simulink model "eovsa_corr_300mhz"  (R2012b)
settings: Solver=VariableStepDiscrete  SolverMode=SingleTasking  StartTime=0.0  StopTime=5000  RelTol=1e-3
undefined symbols (not defined in the file or in its folder): A, B, gcbh, PCIN, sfp, xlBlockLoadCallback, xlipgetpartsetting
libraries: xbsIndex_r4 x5996, casper_library_misc x52, simulink x33, dspsigops x24, xps_library x15, casper_library_delays x2
(part 21 of 65)

== system eovsa_corr_300mhz/pfb_fft/power_td1 ==
  note: The dsp48_sq_add block is a stack of cascaded DSP48 slices.
      | It replaces a previous less efficient implementation that used
      | multipliers followed by an adder tree.  There is more room for
      | optimization here (e.g. by including the accumulation(s) in the
      | stack(s) of cascaded DSP48 slices, but the current (interim)
      | implementation was done to avoid having to change any
      | control logic.
      |
      | The overall latency of the dsp48_sq_add block is 2 cycles
      | longer than the original multipler/adder implementation.
      | To accomodate this change in latency, the sync_in signal
      | has been delayed by a corresponding 2 cycles.
  sync : Inport
  din : Inport  Port=2
  acc_len : Inport  Port=3
  acc_start_skip : Inport  Port=4
  Accumulator2 : xbsIndex_r4/Accumulator  operation=Add  n_bits=48  overflow=Wrap  scale=1  rst=on  infoeditControl=reset for floating point data type must be asserted for a minimum of 2 cycles  hasbypass=off  en=on  latency=0  dbl_ovrd=off  msb_inp=100  msb=100  lsb=-100  use_behavioral_HDL=on  implementation=Fabric  block_type=accum
      settings: block_version=11.4
  Accumulator3 : xbsIndex_r4/Accumulator  operation=Add  n_bits=64  overflow=Wrap  scale=1  rst=on  infoeditControl=reset for floating point data type must be asserted for a minimum of 2 cycles  hasbypass=off  en=on  latency=0  dbl_ovrd=off  msb_inp=100  msb=100  lsb=-100  use_behavioral_HDL=on  implementation=Fabric  block_type=accum
      settings: block_version=11.4
  Accumulator4 : xbsIndex_r4/Accumulator  operation=Add  n_bits=32  overflow=Wrap  scale=1  rst=on  infoeditControl=reset for floating point data type must be asserted for a minimum of 2 cycles  hasbypass=on  en=off  latency=0  dbl_ovrd=off  msb_inp=100  msb=100  lsb=-100  use_behavioral_HDL=off  implementation=DSP48  block_type=accum
      settings: block_version=11.4
  AddSub3 : xbsIndex_r4/AddSub  mode=Addition  use_carryin=off  use_carryout=off  en=off  latency=1  precision=User Defined  arith_type=Unsigned  n_bits=16  bin_pt=0  quantization=Truncate  overflow=Wrap  dbl_ovrd=off  use_behavioral_HDL=on  hw_selection=DSP48  pipelined=off  block_type=addsub
  AddSub4 : xbsIndex_r4/AddSub  mode=Subtraction  use_carryin=off  use_carryout=off  en=off  latency=1  precision=User Defined  arith_type=Unsigned  n_bits=16  bin_pt=0  quantization=Truncate  overflow=Wrap  dbl_ovrd=off  use_behavioral_HDL=on  hw_selection=DSP48  pipelined=off  block_type=addsub
  Constant : xbsIndex_r4/Constant  const=0  gui_display_data_type=Fixed-point  arith_type=Unsigned  n_bits=32  bin_pt=14  preci_type=Single  exp_width=8  frac_width=24  explicit_period=on  period=1  equ=P=C  opselect=C  inp2=PCIN>>17  opr=+  inp1=P  carry=CIN  dbl_ovrd=off  block_type=constant
      settings: block_version=11.4
  Constant1 : xbsIndex_r4/Constant  const=1  gui_display_data_type=Fixed-point  arith_type=Unsigned  n_bits=1  bin_pt=0  preci_type=Single  exp_width=8  frac_width=24  explicit_period=on  period=1  equ=P=C  opselect=C  inp2=PCIN>>17  opr=+  inp1=P  carry=CIN  dbl_ovrd=off  block_type=constant
      settings: block_version=11.4
  Convert1 : xbsIndex_r4/Convert  gui_display_data_type=Fixed-point  arith_type=Unsigned  n_bits=64  bin_pt=18  float_type=Single  exp_bits=8  fraction_bits=24  quantization=Truncate  overflow=Wrap  en=off  latency=0  dbl_ovrd=off  pipeline=off  block_type=convert
      settings: block_version=11.4
  Convert2 : xbsIndex_r4/Convert  gui_display_data_type=Fixed-point  arith_type=Unsigned  n_bits=64  bin_pt=18  float_type=Single  exp_bits=8  fraction_bits=24  quantization=Truncate  overflow=Wrap  en=off  latency=0  dbl_ovrd=off  pipeline=off  block_type=convert
      settings: block_version=11.4
  Convert3 : xbsIndex_r4/Convert  gui_display_data_type=Fixed-point  arith_type=Unsigned  n_bits=32  bin_pt=14  float_type=Single  exp_bits=8  fraction_bits=24  quantization=Truncate  overflow=Wrap  en=off  latency=0  dbl_ovrd=off  pipeline=off  block_type=convert
      settings: block_version=11.4
  Convert4 : xbsIndex_r4/Convert  gui_display_data_type=Fixed-point  arith_type=Unsigned  n_bits=1  bin_pt=0  float_type=Single  exp_bits=8  fraction_bits=24  quantization=Truncate  overflow=Wrap  en=off  latency=0  dbl_ovrd=off  pipeline=off  block_type=convert
      settings: block_version=11.4
  Convert5 : xbsIndex_r4/Convert  gui_display_data_type=Fixed-point  arith_type="Signed  (2's comp)"  n_bits=34  bin_pt=14  float_type=Single  exp_bits=8  fraction_bits=24  quantization=Truncate  overflow=Wrap  en=off  latency=0  dbl_ovrd=off  pipeline=on  block_type=convert
      settings: block_version=11.4
  Counter : xbsIndex_r4/Counter  cnt_type=Free Running  cnt_to=0  operation=Up  start_count=0  cnt_by_val=1  arith_type=Unsigned  n_bits=16  bin_pt=0  load_pin=off  rst=on  en=on  explicit_period=off  period=1  dbl_ovrd=off  use_behavioral_HDL=off  implementation=Fabric  block_type=counter
      settings: block_version=11.4
  Counter1 : xbsIndex_r4/Counter  cnt_type=Free Running  cnt_to=3000  operation=Up  start_count=0  cnt_by_val=1  arith_type=Unsigned  n_bits=32  bin_pt=0  load_pin=off  rst=off  en=on  explicit_period=on  period=1  dbl_ovrd=off  use_behavioral_HDL=on  implementation=Fabric  block_type=counter
      settings: block_version=11.4
  Delay{1,6,9,23} (4 alike) : xbsIndex_r4/Delay  rst=off  infoeditControl=Selection of Reset will increase slice count due to use of real FFs and instead of SRLs  en=off  latency=5  dbl_ovrd=off  reg_retiming=on  block_type=delay
      settings: block_version=11.4
  Delay{2..4,8,10..14,16,18,22,25} (13 alike) : xbsIndex_r4/Delay  rst=off  infoeditControl=Selection of Reset will increase slice count due to use of real FFs and instead of SRLs  en=off  latency=1  dbl_ovrd=off  reg_retiming=on  block_type=delay
      settings: block_version=11.4
  Delay15 : xbsIndex_r4/Delay  rst=off  infoeditControl=Selection of Reset will increase slice count due to use of real FFs and instead of SRLs  en=off  latency=1  dbl_ovrd=off  reg_retiming=off  block_type=delay
      settings: block_version=11.4
  Delay{7,17,19..21} (5 alike) : xbsIndex_r4/Delay  rst=off  infoeditControl=Selection of Reset will increase slice count due to use of real FFs and instead of SRLs  en=off  latency=2  dbl_ovrd=off  reg_retiming=on  block_type=delay
      settings: block_version=11.4
  Delay24 : xbsIndex_r4/Delay  rst=off  infoeditControl=Selection of Reset will increase slice count due to use of real FFs and instead of SRLs  en=off  latency=9  dbl_ovrd=off  reg_retiming=on  block_type=delay
      settings: block_version=11.4
  Delay5 : xbsIndex_r4/Delay  rst=off  infoeditControl=Selection of Reset will increase slice count due to use of real FFs and instead of SRLs  en=off  latency=3  dbl_ovrd=off  reg_retiming=on  block_type=delay
      settings: block_version=11.4
  Logical1 : xbsIndex_r4/Logical  logical_function=XOR  inputs=2  en=off  latency=1  precision=Full  arith_type=Unsigned  n_bits=16  bin_pt=0  align_bp=on  dbl_ovrd=off  block_type=logical
      settings: block_version=11.4
  Mux : xbsIndex_r4/Mux  inputs=2  en=off  latency=1  precision=Full  arith_type=Unsigned  n_bits=16  bin_pt=14  quantization=Truncate  overflow=Wrap  dbl_ovrd=off  block_type=mux
      settings: block_version=11.4
  Reinterpret : xbsIndex_r4/Reinterpret  force_arith_type=on  arith_type=Unsigned  force_bin_pt=on  bin_pt=0  block_type=reinterpret
      settings: infoedit="Changes signal type without altering the binary representation.   You can changed the signal between signed and unsigned, and relocate the binary point.<br><br>Hardware notes: In hardware this block costs nothing.<br><br>Example:  Suppose the input is 6 bits wide, signed, with 2 fractional bits, and the output is forced to unsigned with 0 fractional bits.  Then an input of -2.0 (1110.00 in binary 2's complement) becomes an output of 56 (111000 in binary)."
  Reinterpret1 : xbsIndex_r4/Reinterpret  force_arith_type=on  arith_type=Unsigned  force_bin_pt=on  bin_pt=0  block_type=reinterpret
      settings: infoedit="Changes signal type without altering the binary representation.   You can changed the signal between signed and unsigned, and relocate the binary point.<br><br>Hardware notes: In hardware this block costs nothing.<br><br>Example:  Suppose the input is 6 bits wide, signed, with 2 fractional bits, and the output is forced to unsigned with 0 fractional bits.  Then an input of -2.0 (1110.00 in binary 2's complement) becomes an output of 56 (111000 in binary)."
  Reinterpret2 : xbsIndex_r4/Reinterpret  force_arith_type=on  arith_type=Unsigned  force_bin_pt=on  bin_pt=18  block_type=reinterpret
  Relational2 : xbsIndex_r4/Relational  mode=a<b  en=off  latency=1  dbl_ovrd=off  block_type=relational
  Relational3 : xbsIndex_r4/Relational  mode=a<b  en=off  latency=1  dbl_ovrd=off  block_type=relational
  Slice1 : xbsIndex_r4/Slice  nbits=32  boolean_output=off  mode=Lower Bit Location + Width  bit1=0  base1=MSB of Input  bit0=13  base0=LSB of Input  dbl_ovrd=off  block_type=slice
  big_square_square : Subsystem  AncestorBlock=casper_library_misc/power_dsp48e  mask(wide_power){bitwidth=17}
      mask prompts: bitwidth "Input bit width:"
      mask help: Computes the power of a wide complex number using 3 DSP48Es.
      mask Display:
      | port_label('input', 1, 'c');
      | port_label('output', 1, 'p');
      | disp(['Z^-', num2str(5)]);
  bus_expand : Subsystem  AncestorBlock=casper_library_flow_control/bus_expand  mask(bus_expand){mode=divisions of equal size, outputNum=4, outputWidth=8, outputBinaryPt=7, outputArithmeticType=1, show_format=off, outputToWorkspace=off, variablePrefix=out, outputToModelAsWell=on}
      mask prompts: outputNum "Number of outputs:"; outputWidth "Output width:"; outputBinaryPt "Output binary point position:"; outputArithmeticType "Output arithmetic type (ufix=0, fix=1, bool=2):"; show_format "Print format string?"; outputToWorkspace "Output to workspace?"; variablePrefix "Variable name prefix:"; outputToModelAsWell "Output to model as well?"
      mask help:
      | Expands a 'bus' made using a bus_create or Xilinx
      | concat block.
      | The input will be divided into the specified number
      | of outputs with the specified arithmetic types.
      | Divisions are made from most significant bit.
      mask init: same as eovsa_corr_300mhz/bus_expand7
      settings: AttributesFormatString=4 outputs
      mask TypeOptions mode: divisions of equal size | divisions of arbitrary size
      mask Callback mode: bus_expand_callback();
      mask Callback outputWidth: bus_expand_callback();
      mask Callback outputToWorkspace: bus_expand_callback();
  dsp48_sq_add : Subsystem
  gen_50_pps : Subsystem  mask{fpga_clk_sub=fpga_clk}
      mask prompts: fpga_clk_sub "FPGA Clock Frequency (MHz)"
  pulse generator skip first : Subsystem  mask{period=2 ^ (fft_size - 1)}
      mask prompts: period "Period (clock cycles)"
  acc_num : Outport
  P : Outport  Port=2
  P2 : Outport  Port=3
  acc_valid : Outport  Port=4
  wires:
  sync/1 -> Delay13/1
  Delay14/1 -> dsp48_sq_add/4(d)
  Delay12/1 -> dsp48_sq_add/3(c)
  Delay11/1 -> dsp48_sq_add/2(b)
  Delay10/1 -> dsp48_sq_add/1(a)
  Constant1/1 -> AddSub4/2
  acc_start_skip/1 -> AddSub4/1
  gen_50_pps/2(sync_out) -> pulse generator skip first/1(sync)
  Delay13/1 -> gen_50_pps/1(sync)
  gen_50_pps/1(50pps) -> [pps50]
  Delay9/1 -> Accumulator3/3, Accumulator2/3
  Delay23/1 -> Counter1/1, Delay21/1, Accumulator3/2, Accumulator2/2
  Delay24/1 -> Delay23/1
  Delay22/1 -> Delay9/1
  Delay21/1 -> acc_valid/1
  Delay20/1 -> P2/1
  Delay19/1 -> P/1
  Delay7/1 -> acc_num/1
  Delay18/1 -> Delay22/1
  Delay17/1 -> Delay24/1
  Delay16/1 -> Delay1/1
  [pps50] -> Counter/1
  Accumulator3/1 -> Reinterpret1/1
  Convert1/1 -> Accumulator3/1
  big_square_square/1(p) -> Reinterpret2/1
  Slice1/1 -> Delay19/1
  Reinterpret/1 -> Slice1/1
  Convert2/1 -> Accumulator2/1
  [data_valid] -> Delay18/1
  [data] -> Delay15/1, Delay16/1
  Delay6/1 -> Delay8/1, Accumulator4/2
  Delay4/1 -> Delay5/1
  Convert3/1 -> Delay3/1
  Delay2/1 -> Delay6/1
  [reset_frame] -> Delay25/1
  AddSub4/1 -> Relational3/2, AddSub3/1
  Logical1/1 -> Convert4/1
  [data_frame] -> Mux/3
  Constant/1 -> Mux/2
  Convert4/1 -> Delay4/1
  Relational2/1 -> Logical1/2
  Relational3/1 -> Logical1/1
  AddSub3/1 -> Relational2/2
  acc_len/1 -> AddSub3/2
  Counter/1 -> Relational2/1, Relational3/1
  pulse generator skip first/1(pulse) -> [reset_frame], Counter/2
  [pps50] -> Delay17/1
  Delay1/1 -> Convert2/1
  Reinterpret1/1 -> Delay20/1
  Accumulator2/1 -> Reinterpret/1
  Counter1/1 -> Delay7/1
  dsp48_sq_add/1(p) -> Convert3/1
  bus_expand/3(out2) -> Delay12/1
  bus_expand/2(out3) -> Delay11/1
  bus_expand/1(msb_out4) -> Delay10/1
  bus_expand/4(lsb_out1) -> Delay14/1
  din/1 -> bus_expand/1(bus_in)
  Mux/1 -> [data]
  Delay15/1 -> Convert5/1
  Convert5/1 -> big_square_square/1(c)
  Reinterpret2/1 -> Convert1/1
  Delay8/1 -> [data_valid]
  Accumulator4/1 -> [data_frame]
  Delay5/1 -> Mux/1
  Delay3/1 -> Accumulator4/1
  Delay25/1 -> Delay2/1

== system eovsa_corr_300mhz/pfb_fft/power_td2 ==
  note: The dsp48_sq_add block is a stack of cascaded DSP48 slices.
      | It replaces a previous less efficient implementation that used
      | multipliers followed by an adder tree.  There is more room for
      | optimization here (e.g. by including the accumulation(s) in the
      | stack(s) of cascaded DSP48 slices, but the current (interim)
      | implementation was done to avoid having to change any
      | control logic.
      |
      | The overall latency of the dsp48_sq_add block is 2 cycles
      | longer than the original multipler/adder implementation.
      | To accomodate this change in latency, the sync_in signal
      | has been delayed by a corresponding 2 cycles.
  sync : Inport
  din : Inport  Port=2
  acc_len : Inport  Port=3
  acc_start_skip : Inport  Port=4
  Accumulator2 : xbsIndex_r4/Accumulator  operation=Add  n_bits=48  overflow=Wrap  scale=1  rst=on  infoeditControl=reset for floating point data type must be asserted for a minimum of 2 cycles  hasbypass=off  en=on  latency=0  dbl_ovrd=off  msb_inp=100  msb=100  lsb=-100  use_behavioral_HDL=on  implementation=Fabric  block_type=accum
      settings: block_version=11.4
  Accumulator3 : xbsIndex_r4/Accumulator  operation=Add  n_bits=64  overflow=Wrap  scale=1  rst=on  infoeditControl=reset for floating point data type must be asserted for a minimum of 2 cycles  hasbypass=off  en=on  latency=0  dbl_ovrd=off  msb_inp=100  msb=100  lsb=-100  use_behavioral_HDL=on  implementation=Fabric  block_type=accum
      settings: block_version=11.4
  Accumulator4 : xbsIndex_r4/Accumulator  operation=Add  n_bits=32  overflow=Wrap  scale=1  rst=on  infoeditControl=reset for floating point data type must be asserted for a minimum of 2 cycles  hasbypass=on  en=off  latency=0  dbl_ovrd=off  msb_inp=100  msb=100  lsb=-100  use_behavioral_HDL=off  implementation=DSP48  block_type=accum
      settings: block_version=11.4
  AddSub3 : xbsIndex_r4/AddSub  mode=Addition  use_carryin=off  use_carryout=off  en=off  latency=1  precision=User Defined  arith_type=Unsigned  n_bits=16  bin_pt=0  quantization=Truncate  overflow=Wrap  dbl_ovrd=off  use_behavioral_HDL=on  hw_selection=DSP48  pipelined=off  block_type=addsub
  AddSub4 : xbsIndex_r4/AddSub  mode=Subtraction  use_carryin=off  use_carryout=off  en=off  latency=1  precision=User Defined  arith_type=Unsigned  n_bits=16  bin_pt=0  quantization=Truncate  overflow=Wrap  dbl_ovrd=off  use_behavioral_HDL=on  hw_selection=DSP48  pipelined=off  block_type=addsub
  Constant : xbsIndex_r4/Constant  const=0  gui_display_data_type=Fixed-point  arith_type=Unsigned  n_bits=32  bin_pt=14  preci_type=Single  exp_width=8  frac_width=24  explicit_period=on  period=1  equ=P=C  opselect=C  inp2=PCIN>>17  opr=+  inp1=P  carry=CIN  dbl_ovrd=off  block_type=constant
      settings: block_version=11.4
  Constant1 : xbsIndex_r4/Constant  const=1  gui_display_data_type=Fixed-point  arith_type=Unsigned  n_bits=1  bin_pt=0  preci_type=Single  exp_width=8  frac_width=24  explicit_period=on  period=1  equ=P=C  opselect=C  inp2=PCIN>>17  opr=+  inp1=P  carry=CIN  dbl_ovrd=off  block_type=constant
      settings: block_version=11.4
  Convert1 : xbsIndex_r4/Convert  gui_display_data_type=Fixed-point  arith_type=Unsigned  n_bits=64  bin_pt=18  float_type=Single  exp_bits=8  fraction_bits=24  quantization=Truncate  overflow=Wrap  en=off  latency=0  dbl_ovrd=off  pipeline=off  block_type=convert
      settings: block_version=11.4
  Convert2 : xbsIndex_r4/Convert  gui_display_data_type=Fixed-point  arith_type=Unsigned  n_bits=64  bin_pt=18  float_type=Single  exp_bits=8  fraction_bits=24  quantization=Truncate  overflow=Wrap  en=off  latency=0  dbl_ovrd=off  pipeline=off  block_type=convert
      settings: block_version=11.4
  Convert3 : xbsIndex_r4/Convert  gui_display_data_type=Fixed-point  arith_type=Unsigned  n_bits=32  bin_pt=14  float_type=Single  exp_bits=8  fraction_bits=24  quantization=Truncate  overflow=Wrap  en=off  latency=0  dbl_ovrd=off  pipeline=off  block_type=convert
      settings: block_version=11.4
  Convert4 : xbsIndex_r4/Convert  gui_display_data_type=Fixed-point  arith_type=Unsigned  n_bits=1  bin_pt=0  float_type=Single  exp_bits=8  fraction_bits=24  quantization=Truncate  overflow=Wrap  en=off  latency=0  dbl_ovrd=off  pipeline=off  block_type=convert
      settings: block_version=11.4
  Convert5 : xbsIndex_r4/Convert  gui_display_data_type=Fixed-point  arith_type="Signed  (2's comp)"  n_bits=34  bin_pt=14  float_type=Single  exp_bits=8  fraction_bits=24  quantization=Truncate  overflow=Wrap  en=off  latency=0  dbl_ovrd=off  pipeline=on  block_type=convert
      settings: block_version=11.4
  Counter : xbsIndex_r4/Counter  cnt_type=Free Running  cnt_to=0  operation=Up  start_count=0  cnt_by_val=1  arith_type=Unsigned  n_bits=16  bin_pt=0  load_pin=off  rst=on  en=on  explicit_period=off  period=1  dbl_ovrd=off  use_behavioral_HDL=off  implementation=Fabric  block_type=counter
      settings: block_version=11.4
  Counter1 : xbsIndex_r4/Counter  cnt_type=Free Running  cnt_to=3000  operation=Up  start_count=0  cnt_by_val=1  arith_type=Unsigned  n_bits=32  bin_pt=0  load_pin=off  rst=off  en=on  explicit_period=on  period=1  dbl_ovrd=off  use_behavioral_HDL=on  implementation=Fabric  block_type=counter
      settings: block_version=11.4
  Delay{1,6,9,23} (4 alike) : xbsIndex_r4/Delay  rst=off  infoeditControl=Selection of Reset will increase slice count due to use of real FFs and instead of SRLs  en=off  latency=5  dbl_ovrd=off  reg_retiming=on  block_type=delay
      settings: block_version=11.4
  Delay{2..4,8,10..14,16,18,22,25} (13 alike) : xbsIndex_r4/Delay  rst=off  infoeditControl=Selection of Reset will increase slice count due to use of real FFs and instead of SRLs  en=off  latency=1  dbl_ovrd=off  reg_retiming=on  block_type=delay
      settings: block_version=11.4
  Delay15 : xbsIndex_r4/Delay  rst=off  infoeditControl=Selection of Reset will increase slice count due to use of real FFs and instead of SRLs  en=off  latency=1  dbl_ovrd=off  reg_retiming=off  block_type=delay
      settings: block_version=11.4
  Delay{7,17,19..21} (5 alike) : xbsIndex_r4/Delay  rst=off  infoeditControl=Selection of Reset will increase slice count due to use of real FFs and instead of SRLs  en=off  latency=2  dbl_ovrd=off  reg_retiming=on  block_type=delay
      settings: block_version=11.4
  Delay24 : xbsIndex_r4/Delay  rst=off  infoeditControl=Selection of Reset will increase slice count due to use of real FFs and instead of SRLs  en=off  latency=9  dbl_ovrd=off  reg_retiming=on  block_type=delay
      settings: block_version=11.4
  Delay5 : xbsIndex_r4/Delay  rst=off  infoeditControl=Selection of Reset will increase slice count due to use of real FFs and instead of SRLs  en=off  latency=3  dbl_ovrd=off  reg_retiming=on  block_type=delay
      settings: block_version=11.4
  Logical1 : xbsIndex_r4/Logical  logical_function=XOR  inputs=2  en=off  latency=1  precision=Full  arith_type=Unsigned  n_bits=16  bin_pt=0  align_bp=on  dbl_ovrd=off  block_type=logical
      settings: block_version=11.4
  Mux : xbsIndex_r4/Mux  inputs=2  en=off  latency=1  precision=Full  arith_type=Unsigned  n_bits=16  bin_pt=14  quantization=Truncate  overflow=Wrap  dbl_ovrd=off  block_type=mux
      settings: block_version=11.4
  Reinterpret : xbsIndex_r4/Reinterpret  force_arith_type=on  arith_type=Unsigned  force_bin_pt=on  bin_pt=0  block_type=reinterpret
      settings: infoedit="Changes signal type without altering the binary representation.   You can changed the signal between signed and unsigned, and relocate the binary point.<br><br>Hardware notes: In hardware this block costs nothing.<br><br>Example:  Suppose the input is 6 bits wide, signed, with 2 fractional bits, and the output is forced to unsigned with 0 fractional bits.  Then an input of -2.0 (1110.00 in binary 2's complement) becomes an output of 56 (111000 in binary)."
  Reinterpret1 : xbsIndex_r4/Reinterpret  force_arith_type=on  arith_type=Unsigned  force_bin_pt=on  bin_pt=0  block_type=reinterpret
      settings: infoedit="Changes signal type without altering the binary representation.   You can changed the signal between signed and unsigned, and relocate the binary point.<br><br>Hardware notes: In hardware this block costs nothing.<br><br>Example:  Suppose the input is 6 bits wide, signed, with 2 fractional bits, and the output is forced to unsigned with 0 fractional bits.  Then an input of -2.0 (1110.00 in binary 2's complement) becomes an output of 56 (111000 in binary)."
  Reinterpret2 : xbsIndex_r4/Reinterpret  force_arith_type=on  arith_type=Unsigned  force_bin_pt=on  bin_pt=18  block_type=reinterpret
  Relational2 : xbsIndex_r4/Relational  mode=a<b  en=off  latency=1  dbl_ovrd=off  block_type=relational
  Relational3 : xbsIndex_r4/Relational  mode=a<b  en=off  latency=1  dbl_ovrd=off  block_type=relational
  Slice1 : xbsIndex_r4/Slice  nbits=32  boolean_output=off  mode=Lower Bit Location + Width  bit1=0  base1=MSB of Input  bit0=13  base0=LSB of Input  dbl_ovrd=off  block_type=slice
  big_square_square : Subsystem  AncestorBlock=casper_library_misc/power_dsp48e  mask(wide_power){bitwidth=17}
      mask prompts: bitwidth "Input bit width:"
      mask help: Computes the power of a wide complex number using 3 DSP48Es.
      mask Display:
      | port_label('input', 1, 'c');
      | port_label('output', 1, 'p');
      | disp(['Z^-', num2str(5)]);
  bus_expand : Subsystem  AncestorBlock=casper_library_flow_control/bus_expand  mask(bus_expand){mode=divisions of equal size, outputNum=4, outputWidth=8, outputBinaryPt=7, outputArithmeticType=1, show_format=off, outputToWorkspace=off, variablePrefix=out, outputToModelAsWell=on}
      mask prompts: outputNum "Number of outputs:"; outputWidth "Output width:"; outputBinaryPt "Output binary point position:"; outputArithmeticType "Output arithmetic type (ufix=0, fix=1, bool=2):"; show_format "Print format string?"; outputToWorkspace "Output to workspace?"; variablePrefix "Variable name prefix:"; outputToModelAsWell "Output to model as well?"
      mask help:
      | Expands a 'bus' made using a bus_create or Xilinx
      | concat block.
      | The input will be divided into the specified number
      | of outputs with the specified arithmetic types.
      | Divisions are made from most significant bit.
      mask init: same as eovsa_corr_300mhz/bus_expand7
      settings: AttributesFormatString=4 outputs
      mask TypeOptions mode: divisions of equal size | divisions of arbitrary size
      mask Callback mode: bus_expand_callback();
      mask Callback outputWidth: bus_expand_callback();
      mask Callback outputToWorkspace: bus_expand_callback();
  dsp48_sq_add : Subsystem
  gen_50_pps : Subsystem  mask{fpga_clk_sub=fpga_clk}
      mask prompts: fpga_clk_sub "FPGA Clock Frequency (MHz)"
  pulse generator skip first : Subsystem  mask{period=2 ^ (fft_size - 1)}
      mask prompts: period "Period (clock cycles)"
  acc_num : Outport
  P : Outport  Port=2
  P2 : Outport  Port=3
  acc_valid : Outport  Port=4
  wires:
  Delay25/1 -> Delay2/1
  Delay3/1 -> Accumulator4/1
  Delay5/1 -> Mux/1
  Accumulator4/1 -> [data_frame]
  Delay8/1 -> [data_valid]
  Reinterpret2/1 -> Convert1/1
  Convert5/1 -> big_square_square/1(c)
  Delay15/1 -> Convert5/1
  Mux/1 -> [data]
  din/1 -> bus_expand/1(bus_in)
  bus_expand/4(lsb_out1) -> Delay14/1
  bus_expand/1(msb_out4) -> Delay10/1
  bus_expand/2(out3) -> Delay11/1
  bus_expand/3(out2) -> Delay12/1
  dsp48_sq_add/1(p) -> Convert3/1
  Counter1/1 -> Delay7/1
  Accumulator2/1 -> Reinterpret/1
  Reinterpret1/1 -> Delay20/1
  Delay1/1 -> Convert2/1
  [pps50] -> Delay17/1
  pulse generator skip first/1(pulse) -> Counter/2, [reset_frame]
  Counter/1 -> Relational3/1, Relational2/1
  acc_len/1 -> AddSub3/2
  AddSub3/1 -> Relational2/2
  Relational3/1 -> Logical1/1
  Relational2/1 -> Logical1/2
  Convert4/1 -> Delay4/1
  Constant/1 -> Mux/2
  [data_frame] -> Mux/3
  Logical1/1 -> Convert4/1
  AddSub4/1 -> AddSub3/1, Relational3/2
  [reset_frame] -> Delay25/1
  Delay2/1 -> Delay6/1
  Convert3/1 -> Delay3/1
  Delay4/1 -> Delay5/1
  Delay6/1 -> Accumulator4/2, Delay8/1
  [data] -> Delay16/1, Delay15/1
  [data_valid] -> Delay18/1
  Convert2/1 -> Accumulator2/1
  Reinterpret/1 -> Slice1/1
  Slice1/1 -> Delay19/1
  big_square_square/1(p) -> Reinterpret2/1
  Convert1/1 -> Accumulator3/1
  Accumulator3/1 -> Reinterpret1/1
  [pps50] -> Counter/1
  Delay16/1 -> Delay1/1
  Delay17/1 -> Delay24/1
  Delay18/1 -> Delay22/1
  Delay7/1 -> acc_num/1
  Delay19/1 -> P/1
  Delay20/1 -> P2/1
  Delay21/1 -> acc_valid/1
  Delay22/1 -> Delay9/1
  Delay24/1 -> Delay23/1
  Delay23/1 -> Accumulator2/2, Accumulator3/2, Delay21/1, Counter1/1
  Delay9/1 -> Accumulator2/3, Accumulator3/3
  gen_50_pps/1(50pps) -> [pps50]
  Delay13/1 -> gen_50_pps/1(sync)
  gen_50_pps/2(sync_out) -> pulse generator skip first/1(sync)
  acc_start_skip/1 -> AddSub4/1
  Constant1/1 -> AddSub4/2
  Delay10/1 -> dsp48_sq_add/1(a)
  Delay11/1 -> dsp48_sq_add/2(b)
  Delay12/1 -> dsp48_sq_add/3(c)
  Delay14/1 -> dsp48_sq_add/4(d)
  sync/1 -> Delay13/1

== system eovsa_corr_300mhz/pfb_fft/power_td3 ==
  note: The dsp48_sq_add block is a stack of cascaded DSP48 slices.
      | It replaces a previous less efficient implementation that used
      | multipliers followed by an adder tree.  There is more room for
      | optimization here (e.g. by including the accumulation(s) in the
      | stack(s) of cascaded DSP48 slices, but the current (interim)
      | implementation was done to avoid having to change any
      | control logic.
      |
      | The overall latency of the dsp48_sq_add block is 2 cycles
      | longer than the original multipler/adder implementation.
      | To accomodate this change in latency, the sync_in signal
      | has been delayed by a corresponding 2 cycles.
  sync : Inport
  din : Inport  Port=2
  acc_len : Inport  Port=3
  acc_start_skip : Inport  Port=4
  Accumulator2 : xbsIndex_r4/Accumulator  operation=Add  n_bits=48  overflow=Wrap  scale=1  rst=on  infoeditControl=reset for floating point data type must be asserted for a minimum of 2 cycles  hasbypass=off  en=on  latency=0  dbl_ovrd=off  msb_inp=100  msb=100  lsb=-100  use_behavioral_HDL=on  implementation=Fabric  block_type=accum
      settings: block_version=11.4
  Accumulator3 : xbsIndex_r4/Accumulator  operation=Add  n_bits=64  overflow=Wrap  scale=1  rst=on  infoeditControl=reset for floating point data type must be asserted for a minimum of 2 cycles  hasbypass=off  en=on  latency=0  dbl_ovrd=off  msb_inp=100  msb=100  lsb=-100  use_behavioral_HDL=on  implementation=Fabric  block_type=accum
      settings: block_version=11.4
  Accumulator4 : xbsIndex_r4/Accumulator  operation=Add  n_bits=32  overflow=Wrap  scale=1  rst=on  infoeditControl=reset for floating point data type must be asserted for a minimum of 2 cycles  hasbypass=on  en=off  latency=0  dbl_ovrd=off  msb_inp=100  msb=100  lsb=-100  use_behavioral_HDL=off  implementation=DSP48  block_type=accum
      settings: block_version=11.4
  AddSub3 : xbsIndex_r4/AddSub  mode=Addition  use_carryin=off  use_carryout=off  en=off  latency=1  precision=User Defined  arith_type=Unsigned  n_bits=16  bin_pt=0  quantization=Truncate  overflow=Wrap  dbl_ovrd=off  use_behavioral_HDL=on  hw_selection=DSP48  pipelined=off  block_type=addsub
  AddSub4 : xbsIndex_r4/AddSub  mode=Subtraction  use_carryin=off  use_carryout=off  en=off  latency=1  precision=User Defined  arith_type=Unsigned  n_bits=16  bin_pt=0  quantization=Truncate  overflow=Wrap  dbl_ovrd=off  use_behavioral_HDL=on  hw_selection=DSP48  pipelined=off  block_type=addsub
  Constant : xbsIndex_r4/Constant  const=0  gui_display_data_type=Fixed-point  arith_type=Unsigned  n_bits=32  bin_pt=14  preci_type=Single  exp_width=8  frac_width=24  explicit_period=on  period=1  equ=P=C  opselect=C  inp2=PCIN>>17  opr=+  inp1=P  carry=CIN  dbl_ovrd=off  block_type=constant
      settings: block_version=11.4
  Constant1 : xbsIndex_r4/Constant  const=1  gui_display_data_type=Fixed-point  arith_type=Unsigned  n_bits=1  bin_pt=0  preci_type=Single  exp_width=8  frac_width=24  explicit_period=on  period=1  equ=P=C  opselect=C  inp2=PCIN>>17  opr=+  inp1=P  carry=CIN  dbl_ovrd=off  block_type=constant
      settings: block_version=11.4
  Convert1 : xbsIndex_r4/Convert  gui_display_data_type=Fixed-point  arith_type=Unsigned  n_bits=64  bin_pt=18  float_type=Single  exp_bits=8  fraction_bits=24  quantization=Truncate  overflow=Wrap  en=off  latency=0  dbl_ovrd=off  pipeline=off  block_type=convert
      settings: block_version=11.4
  Convert2 : xbsIndex_r4/Convert  gui_display_data_type=Fixed-point  arith_type=Unsigned  n_bits=64  bin_pt=18  float_type=Single  exp_bits=8  fraction_bits=24  quantization=Truncate  overflow=Wrap  en=off  latency=0  dbl_ovrd=off  pipeline=off  block_type=convert
      settings: block_version=11.4
  Convert3 : xbsIndex_r4/Convert  gui_display_data_type=Fixed-point  arith_type=Unsigned  n_bits=32  bin_pt=14  float_type=Single  exp_bits=8  fraction_bits=24  quantization=Truncate  overflow=Wrap  en=off  latency=0  dbl_ovrd=off  pipeline=off  block_type=convert
      settings: block_version=11.4
  Convert4 : xbsIndex_r4/Convert  gui_display_data_type=Fixed-point  arith_type=Unsigned  n_bits=1  bin_pt=0  float_type=Single  exp_bits=8  fraction_bits=24  quantization=Truncate  overflow=Wrap  en=off  latency=0  dbl_ovrd=off  pipeline=off  block_type=convert
      settings: block_version=11.4
  Convert5 : xbsIndex_r4/Convert  gui_display_data_type=Fixed-point  arith_type="Signed  (2's comp)"  n_bits=34  bin_pt=14  float_type=Single  exp_bits=8  fraction_bits=24  quantization=Truncate  overflow=Wrap  en=off  latency=0  dbl_ovrd=off  pipeline=on  block_type=convert
      settings: block_version=11.4
  Counter : xbsIndex_r4/Counter  cnt_type=Free Running  cnt_to=0  operation=Up  start_count=0  cnt_by_val=1  arith_type=Unsigned  n_bits=16  bin_pt=0  load_pin=off  rst=on  en=on  explicit_period=off  period=1  dbl_ovrd=off  use_behavioral_HDL=off  implementation=Fabric  block_type=counter
      settings: block_version=11.4
  Counter1 : xbsIndex_r4/Counter  cnt_type=Free Running  cnt_to=3000  operation=Up  start_count=0  cnt_by_val=1  arith_type=Unsigned  n_bits=32  bin_pt=0  load_pin=off  rst=off  en=on  explicit_period=on  period=1  dbl_ovrd=off  use_behavioral_HDL=on  implementation=Fabric  block_type=counter
      settings: block_version=11.4
  Delay{1,6,9,23} (4 alike) : xbsIndex_r4/Delay  rst=off  infoeditControl=Selection of Reset will increase slice count due to use of real FFs and instead of SRLs  en=off  latency=5  dbl_ovrd=off  reg_retiming=on  block_type=delay
      settings: block_version=11.4
  Delay{2..4,8,10..14,16,18,22,25} (13 alike) : xbsIndex_r4/Delay  rst=off  infoeditControl=Selection of Reset will increase slice count due to use of real FFs and instead of SRLs  en=off  latency=1  dbl_ovrd=off  reg_retiming=on  block_type=delay
      settings: block_version=11.4
  Delay15 : xbsIndex_r4/Delay  rst=off  infoeditControl=Selection of Reset will increase slice count due to use of real FFs and instead of SRLs  en=off  latency=1  dbl_ovrd=off  reg_retiming=off  block_type=delay
      settings: block_version=11.4
  Delay{7,17,19..21} (5 alike) : xbsIndex_r4/Delay  rst=off  infoeditControl=Selection of Reset will increase slice count due to use of real FFs and instead of SRLs  en=off  latency=2  dbl_ovrd=off  reg_retiming=on  block_type=delay
      settings: block_version=11.4
  Delay24 : xbsIndex_r4/Delay  rst=off  infoeditControl=Selection of Reset will increase slice count due to use of real FFs and instead of SRLs  en=off  latency=9  dbl_ovrd=off  reg_retiming=on  block_type=delay
      settings: block_version=11.4
  Delay5 : xbsIndex_r4/Delay  rst=off  infoeditControl=Selection of Reset will increase slice count due to use of real FFs and instead of SRLs  en=off  latency=3  dbl_ovrd=off  reg_retiming=on  block_type=delay
      settings: block_version=11.4
  Logical1 : xbsIndex_r4/Logical  logical_function=XOR  inputs=2  en=off  latency=1  precision=Full  arith_type=Unsigned  n_bits=16  bin_pt=0  align_bp=on  dbl_ovrd=off  block_type=logical
      settings: block_version=11.4
  Mux : xbsIndex_r4/Mux  inputs=2  en=off  latency=1  precision=Full  arith_type=Unsigned  n_bits=16  bin_pt=14  quantization=Truncate  overflow=Wrap  dbl_ovrd=off  block_type=mux
      settings: block_version=11.4
  Reinterpret : xbsIndex_r4/Reinterpret  force_arith_type=on  arith_type=Unsigned  force_bin_pt=on  bin_pt=0  block_type=reinterpret
      settings: infoedit="Changes signal type without altering the binary representation.   You can changed the signal between signed and unsigned, and relocate the binary point.<br><br>Hardware notes: In hardware this block costs nothing.<br><br>Example:  Suppose the input is 6 bits wide, signed, with 2 fractional bits, and the output is forced to unsigned with 0 fractional bits.  Then an input of -2.0 (1110.00 in binary 2's complement) becomes an output of 56 (111000 in binary)."
  Reinterpret1 : xbsIndex_r4/Reinterpret  force_arith_type=on  arith_type=Unsigned  force_bin_pt=on  bin_pt=0  block_type=reinterpret
      settings: infoedit="Changes signal type without altering the binary representation.   You can changed the signal between signed and unsigned, and relocate the binary point.<br><br>Hardware notes: In hardware this block costs nothing.<br><br>Example:  Suppose the input is 6 bits wide, signed, with 2 fractional bits, and the output is forced to unsigned with 0 fractional bits.  Then an input of -2.0 (1110.00 in binary 2's complement) becomes an output of 56 (111000 in binary)."
  Reinterpret2 : xbsIndex_r4/Reinterpret  force_arith_type=on  arith_type=Unsigned  force_bin_pt=on  bin_pt=18  block_type=reinterpret
  Relational2 : xbsIndex_r4/Relational  mode=a<b  en=off  latency=1  dbl_ovrd=off  block_type=relational
  Relational3 : xbsIndex_r4/Relational  mode=a<b  en=off  latency=1  dbl_ovrd=off  block_type=relational
  Slice1 : xbsIndex_r4/Slice  nbits=32  boolean_output=off  mode=Lower Bit Location + Width  bit1=0  base1=MSB of Input  bit0=13  base0=LSB of Input  dbl_ovrd=off  block_type=slice
  big_square_square : Subsystem  AncestorBlock=casper_library_misc/power_dsp48e  mask(wide_power){bitwidth=17}
      mask prompts: bitwidth "Input bit width:"
      mask help: Computes the power of a wide complex number using 3 DSP48Es.
      mask Display:
      | port_label('input', 1, 'c');
      | port_label('output', 1, 'p');
      | disp(['Z^-', num2str(5)]);
  bus_expand : Subsystem  AncestorBlock=casper_library_flow_control/bus_expand  mask(bus_expand){mode=divisions of equal size, outputNum=4, outputWidth=8, outputBinaryPt=7, outputArithmeticType=1, show_format=off, outputToWorkspace=off, variablePrefix=out, outputToModelAsWell=on}
      mask prompts: outputNum "Number of outputs:"; outputWidth "Output width:"; outputBinaryPt "Output binary point position:"; outputArithmeticType "Output arithmetic type (ufix=0, fix=1, bool=2):"; show_format "Print format string?"; outputToWorkspace "Output to workspace?"; variablePrefix "Variable name prefix:"; outputToModelAsWell "Output to model as well?"
      mask help:
      | Expands a 'bus' made using a bus_create or Xilinx
      | concat block.
      | The input will be divided into the specified number
      | of outputs with the specified arithmetic types.
      | Divisions are made from most significant bit.
      mask init: same as eovsa_corr_300mhz/bus_expand7
      settings: AttributesFormatString=4 outputs
      mask TypeOptions mode: divisions of equal size | divisions of arbitrary size
      mask Callback mode: bus_expand_callback();
      mask Callback outputWidth: bus_expand_callback();
      mask Callback outputToWorkspace: bus_expand_callback();
  dsp48_sq_add : Subsystem
  gen_50_pps : Subsystem  mask{fpga_clk_sub=fpga_clk}
      mask prompts: fpga_clk_sub "FPGA Clock Frequency (MHz)"
  pulse generator skip first : Subsystem  mask{period=2 ^ (fft_size - 1)}
      mask prompts: period "Period (clock cycles)"
  acc_num : Outport
  P : Outport  Port=2
  P2 : Outport  Port=3
  acc_valid : Outport  Port=4
  wires:
  Delay25/1 -> Delay2/1
  Delay3/1 -> Accumulator4/1
  Delay5/1 -> Mux/1
  Accumulator4/1 -> [data_frame]
  Delay8/1 -> [data_valid]
  Reinterpret2/1 -> Convert1/1
  Convert5/1 -> big_square_square/1(c)
  Delay15/1 -> Convert5/1
  Mux/1 -> [data]
  din/1 -> bus_expand/1(bus_in)
  bus_expand/4(lsb_out1) -> Delay14/1
  bus_expand/1(msb_out4) -> Delay10/1
  bus_expand/2(out3) -> Delay11/1
  bus_expand/3(out2) -> Delay12/1
  dsp48_sq_add/1(p) -> Convert3/1
  Counter1/1 -> Delay7/1
  Accumulator2/1 -> Reinterpret/1
  Reinterpret1/1 -> Delay20/1
  Delay1/1 -> Convert2/1
  [pps50] -> Delay17/1
  pulse generator skip first/1(pulse) -> Counter/2, [reset_frame]
  Counter/1 -> Relational3/1, Relational2/1
  acc_len/1 -> AddSub3/2
  AddSub3/1 -> Relational2/2
  Relational3/1 -> Logical1/1
  Relational2/1 -> Logical1/2
  Convert4/1 -> Delay4/1
  Constant/1 -> Mux/2
  [data_frame] -> Mux/3
  Logical1/1 -> Convert4/1
  AddSub4/1 -> AddSub3/1, Relational3/2
  [reset_frame] -> Delay25/1
  Delay2/1 -> Delay6/1
  Convert3/1 -> Delay3/1
  Delay4/1 -> Delay5/1
  Delay6/1 -> Accumulator4/2, Delay8/1
  [data] -> Delay16/1, Delay15/1
  [data_valid] -> Delay18/1
  Convert2/1 -> Accumulator2/1
  Reinterpret/1 -> Slice1/1
  Slice1/1 -> Delay19/1
  big_square_square/1(p) -> Reinterpret2/1
  Convert1/1 -> Accumulator3/1
  Accumulator3/1 -> Reinterpret1/1
  [pps50] -> Counter/1
  Delay16/1 -> Delay1/1
  Delay17/1 -> Delay24/1
  Delay18/1 -> Delay22/1
  Delay7/1 -> acc_num/1
  Delay19/1 -> P/1
  Delay20/1 -> P2/1
  Delay21/1 -> acc_valid/1
  Delay22/1 -> Delay9/1
  Delay24/1 -> Delay23/1
  Delay23/1 -> Accumulator2/2, Accumulator3/2, Delay21/1, Counter1/1
  Delay9/1 -> Accumulator2/3, Accumulator3/3
  gen_50_pps/1(50pps) -> [pps50]
  Delay13/1 -> gen_50_pps/1(sync)
  gen_50_pps/2(sync_out) -> pulse generator skip first/1(sync)
  acc_start_skip/1 -> AddSub4/1
  Constant1/1 -> AddSub4/2
  Delay10/1 -> dsp48_sq_add/1(a)
  Delay11/1 -> dsp48_sq_add/2(b)
  Delay12/1 -> dsp48_sq_add/3(c)
  Delay14/1 -> dsp48_sq_add/4(d)
  sync/1 -> Delay13/1
